simulink subsystem "GenCtrl"  (R2024b)
settings: Solver=VariableStepAuto  StartTime=0.0  StopTime=10.0  RelTol=1e-3
undefined symbols (not defined in the file or in its folder): SimIn, SimPar
libraries: simulink_extras x7, libAxisTransformations x3, ComponentsLib x3
settings Model: Creator=tbritton  LastModifiedBy=mjki1
settings SolverCC: AlgebraicLoopSolver=TrustRegion
settings OptimizationCC: ReuseModelBlockBuffer=off
settings DebuggingCC: UnconnectedInputMsg=warning  UnconnectedOutputMsg=warning  UnconnectedLineMsg=warning
settings ModelReferenceCC: EnableRefExpFcnMdlSchedulingChecks=on
settings RTWCC: GPUComputeCapability=3.5  DLArmComputeVersion=19.05

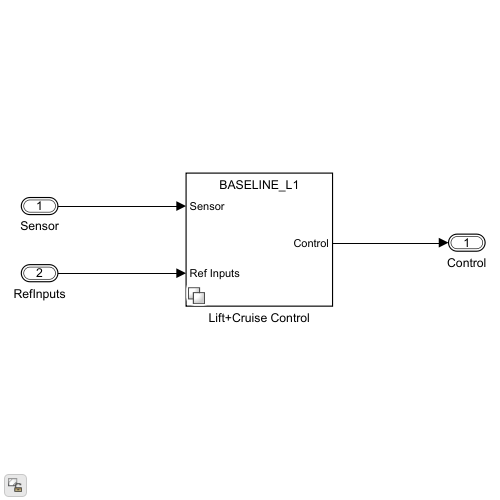
[thumbnail: Simulink's stored preview of the top-level diagram]
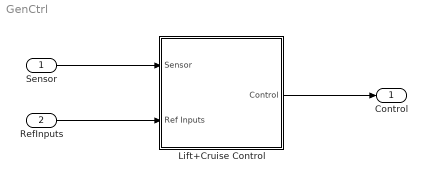
== system GenCtrl ==
  Sensor : Inport  OutDataTypeStr=Bus: SensorBus
  RefInputs : Inport  Port=2  OutDataTypeStr=Bus: BUS_REF_INPUT
  Lift+Cruise Control : Subsystem  Variant=on
  Control : Outport  OutDataTypeStr=Bus: BUS_CONTROL
  wires:
  Sensor/1 -> Lift+Cruise Control/1(Sensor)
  RefInputs/1 -> Lift+Cruise Control/2(Ref Inputs)
  Lift+Cruise Control/1(Control) -> Control/1

== system GenCtrl/Lift+Cruise Control ==
  Sensor : Inport  OutDataTypeStr=Bus: SensorBus
  Ref Inputs : Inport  Port=2  OutDataTypeStr=Bus: BUS_REF_INPUT
  BASELINE : Subsystem  VariantControl=GVS_CTRL_TYPE_BASELINE  ReferencedSubsystem=Baseline
  BASELINE_AGI : Subsystem  VariantControl=GVS_CTRL_TYPE_BASELINE_AGI  ReferencedSubsystem=BASELINE_AGI
  BASELINE_L1 : Subsystem  VariantControl=GVS_CTRL_TYPE_BASELINE_L1
  TRIM : Subsystem  VariantControl=GVS_CTRL_TYPE_TRIM  ReferencedSubsystem=TRIM
  Control : Outport  OutDataTypeStr=Bus: BUS_CONTROL  VectorParamsAs1DForOutWhenUnconnected=off

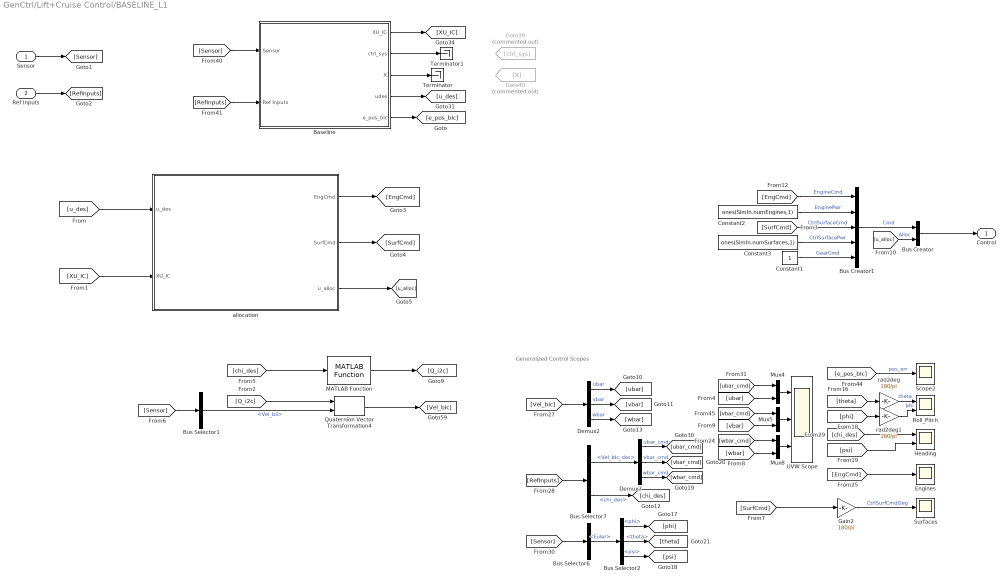
== system GenCtrl/Lift+Cruise Control/BASELINE_L1 ==
  note: Generalized Control Scopes
  Sensor : Inport  OutDataTypeStr=Bus: SensorBus
  Ref Inputs : Inport  Port=2  OutDataTypeStr=Bus: BUS_REF_INPUT
  Baseline : Subsystem
      settings: LibrarySourceBlock=ControllersLib/Baseline
  Bus Creator : BusCreator  Inputs=2
  Bus Creator1 : BusCreator  Inputs=5  OutDataTypeStr=Bus: BUS_CMD
  Bus Selector1 : BusSelector  OutputSignals=Vel_bIi
  Bus Selector2 : BusSelector  OutputSignals=phi,theta,psi
  Bus Selector6 : BusSelector  OutputSignals=Euler
  Bus Selector7 : BusSelector  OutputSignals=Vel_bIc_des,chi_des
  Constant1 : Constant
  Constant2 : Constant  Value=ones(SimIn.numEngines,1)
  Constant3 : Constant  Value=ones(SimIn.numSurfaces,1)
  Demux2 : Demux  Outputs=3
  Demux3 : Demux  Outputs=3
  Engines : Scope
  Gain2 : Gain  Gain=180/pi
  Goto39 : Goto  Commented=on  GotoTag=ctrl_sys
  Goto40 : Goto  Commented=on  GotoTag=X
  Heading : Scope  NumInputPorts=2
  MATLAB Function : ComponentsLib/ConvertToControlFrame/MATLAB Function  SystemSampleTime=-1  VariantActivationTime=update diagram  AllowFlexibleInterface=on  Latency=0  AutoFrameSizeCalculation=off
      settings: SourceProductName=Components
  Mux4 : Mux  Inputs=2
  Mux5 : Mux  Inputs=2
  Mux8 : Mux  Inputs=2
  Quaternion Vector Transformation4 : libAxisTransformations/Quaternion Vector Transformation  n=0
  Roll_Pitch : Scope  NumInputPorts=2
  Scope2 : Scope
  Surfaces : Scope
  Terminator : Terminator
  Terminator1 : Terminator
  UVW Scope : Scope  NumInputPorts=3
  allocation : Subsystem
  rad2deg : Gain  Gain=180/pi
  rad2deg1 : Gain  Gain=180/pi
  Control : Outport  OutDataTypeStr=Bus: BUS_CONTROL  VectorParamsAs1DForOutWhenUnconnected=off
  wires:
  Bus Creator/1 -> Control/1
  [u_alloc] -> Bus Creator/2  "Alloc"
  allocation/3(u_alloc) -> [u_alloc]
  allocation/2(SurfCmd) -> [SurfCmd]
  allocation/1(EngCmd) -> [EngCmd]
  [u_des] -> allocation/1(u_des)
  [XU_IC] -> allocation/2(XU_IC)
  [SurfCmd] -> Bus Creator1/3  "CtrlSurfaceCmd"
  Bus Creator1/1 -> Bus Creator/1  "Cmd"
  Constant3/1 -> Bus Creator1/4  "CtrlSurfacePwr"
  Constant1/1 -> Bus Creator1/5  "GearCmd"
  Constant2/1 -> Bus Creator1/2  "EnginePwr"
  [EngCmd] -> Bus Creator1/1  "EngineCmd"
  Baseline/1(XU_IC) -> [XU_IC]
  Baseline/5(e_pos_blc) -> [e_pos_bIc]
  Baseline/3(X) -> Terminator/1
  [Sensor] -> Baseline/1(Sensor)
  [RefInputs] -> Baseline/2(Ref Inputs)
  Baseline/4(udes) -> [u_des]
  Baseline/2(ctrl_sys) -> Terminator1/1
  Sensor/1 -> [Sensor]
  Ref Inputs/1 -> [RefInputs]
  MATLAB Function/1 -> [Q_i2c]
  Quaternion Vector Transformation4/1 -> [Vel_bIc]
  [Sensor] -> Bus Selector1/1
  Bus Selector1/1 -> Quaternion Vector Transformation4/2  "<Vel_bIi>"
  [Q_i2c] -> Quaternion Vector Transformation4/1
  [chi_des] -> MATLAB Function/1
  Demux3/2 -> [vbar_cmd]  "vbar_cmd"
  [Sensor] -> Bus Selector6/1
  Bus Selector7/1 -> Demux3/1  "<Vel_bIc_des>"
  Bus Selector2/2 -> [theta]  "<theta>"
  rad2deg/1 -> Roll_Pitch/1  "theta"
  [ubar_cmd] -> Mux4/1
  Mux4/1 -> UVW Scope/1
  Bus Selector6/1 -> Bus Selector2/1  "<Euler>"
  [e_pos_bIc] -> Scope2/1  "pos_err"
  Demux2/2 -> [vbar]  "vbar"
  [vbar] -> Mux5/2
  [wbar_cmd] -> Mux8/1
  [psi] -> Heading/2
  [phi] -> rad2deg1/1
  Bus Selector2/3 -> [psi]  "<psi>"
  Bus Selector7/2 -> [chi_des]  "<chi_des>"
  Mux5/1 -> UVW Scope/2
  Demux2/1 -> [ubar]  "ubar"
  Gain2/1 -> Surfaces/1  "CtrlSurfCmdDeg"
  [Vel_bIc] -> Demux2/1
  [wbar] -> Mux8/2
  [chi_des] -> Heading/1
  Demux2/3 -> [wbar]  "wbar"
  Mux8/1 -> UVW Scope/3
  [EngCmd] -> Engines/1
  [vbar_cmd] -> Mux5/1
  Demux3/3 -> [wbar_cmd]  "wbar_cmd"
  [SurfCmd] -> Gain2/1
  [ubar] -> Mux4/2
  Demux3/1 -> [ubar_cmd]  "ubar_cmd"
  rad2deg1/1 -> Roll_Pitch/2  "phi"
  [RefInputs] -> Bus Selector7/1
  Bus Selector2/1 -> [phi]  "<phi>"
  [theta] -> rad2deg/1

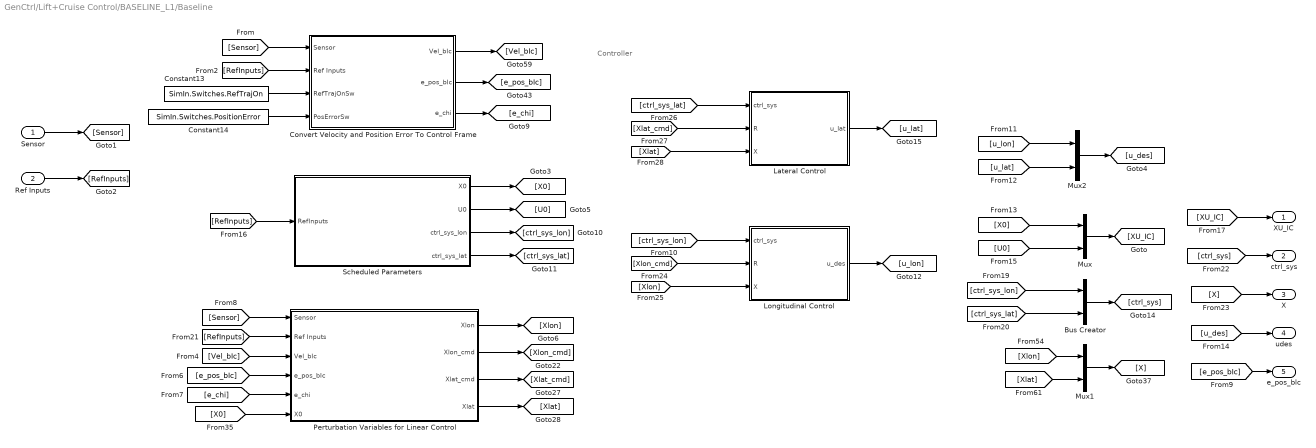
== system GenCtrl/Lift+Cruise Control/BASELINE_L1/Baseline ==
  note: Controller
  Sensor : Inport  OutDataTypeStr=Bus: SensorBus
  Ref Inputs : Inport  Port=2  OutDataTypeStr=Bus: BUS_REF_INPUT
  Bus Creator : BusCreator  Inputs=2
  Constant13 : Constant  Value=SimIn.Switches.RefTrajOn
  Constant14 : Constant  Value=SimIn.Switches.PositionError
  Convert Velocity and Position Error To Control Frame : Subsystem  AncestorBlock=ComponentsLib/ConvertToControlFrame
  Lateral Control : Subsystem
  Longitudinal Control : Subsystem
  Mux : Mux  Inputs=2
  Mux1 : Mux  Inputs=2
  Mux2 : Mux  Inputs=2
  Perturbation Variables for Linear Control : Subsystem  AncestorBlock=ComponentsLib/ComputePerturbationVariables
  Scheduled Parameters : Subsystem  AncestorBlock=ComponentsLib/FeedbackScheduling
      settings: LibrarySourceBlock=ComponentsLib/FeedbackScheduling
  XU_IC : Outport
  ctrl_sys : Outport  Port=2
  X : Outport  Port=3
  udes : Outport  Port=4
  e_pos_blc : Outport  Port=5
  wires:
  Mux2/1 -> [u_des]
  [u_lat] -> Mux2/2
  [u_lon] -> Mux2/1
  [e_pos_bIc] -> e_pos_blc/1
  [X0] -> Perturbation Variables for Linear Control/6(X0)
  Perturbation Variables for Linear Control/1(Xlon) -> [Xlon]
  [Sensor] -> Perturbation Variables for Linear Control/1(Sensor)
  Perturbation Variables for Linear Control/3(Xlat_cmd) -> [Xlat_cmd]
  Sensor/1 -> [Sensor]
  Scheduled Parameters/1(X0) -> [X0]
  Ref Inputs/1 -> [RefInputs]
  [RefInputs] -> Convert Velocity and Position Error To Control Frame/2(Ref Inputs)
  Convert Velocity and Position Error To Control Frame/1(Vel_bIc) -> [Vel_bIc]
  Convert Velocity and Position Error To Control Frame/2(e_pos_bIc) -> [e_pos_bIc]
  Scheduled Parameters/3(ctrl_sys_lon) -> [ctrl_sys_lon]
  [e_pos_bIc] -> Perturbation Variables for Linear Control/4(e_pos_bIc)
  Perturbation Variables for Linear Control/4(Xlat) -> [Xlat]
  [RefInputs] -> Scheduled Parameters/1(RefInputs)
  Perturbation Variables for Linear Control/2(Xlon_cmd) -> [Xlon_cmd]
  Convert Velocity and Position Error To Control Frame/3(e_chi) -> [e_chi]
  [Sensor] -> Convert Velocity and Position Error To Control Frame/1(Sensor)
  [Vel_bIc] -> Perturbation Variables for Linear Control/3(Vel_bIc)
  Constant13/1 -> Convert Velocity and Position Error To Control Frame/3(RefTrajOnSw)
  [RefInputs] -> Perturbation Variables for Linear Control/2(Ref Inputs)
  Constant14/1 -> Convert Velocity and Position Error To Control Frame/4(PosErrorSw)
  [e_chi] -> Perturbation Variables for Linear Control/5(e_chi)
  Scheduled Parameters/2(U0) -> [U0]
  Scheduled Parameters/4(ctrl_sys_lat) -> [ctrl_sys_lat]
  [u_des] -> udes/1
  [X0] -> Mux/1
  [U0] -> Mux/2
  Mux/1 -> [XU_IC]
  [XU_IC] -> XU_IC/1
  [ctrl_sys_lon] -> Bus Creator/1
  [ctrl_sys_lat] -> Bus Creator/2
  Bus Creator/1 -> [ctrl_sys]
  [ctrl_sys] -> ctrl_sys/1
  Mux1/1 -> [X]
  [Xlon] -> Mux1/1
  [Xlat] -> Mux1/2
  [X] -> X/1
  [ctrl_sys_lon] -> Longitudinal Control/1(ctrl_sys)
  [Xlon_cmd] -> Longitudinal Control/2(R)
  [Xlon] -> Longitudinal Control/3(X)
  Longitudinal Control/1(u_des) -> [u_lon]
  Lateral Control/1(u_lat) -> [u_lat]
  [Xlat_cmd] -> Lateral Control/2(R)
  [Xlat] -> Lateral Control/3(X)
  [ctrl_sys_lat] -> Lateral Control/1(ctrl_sys)

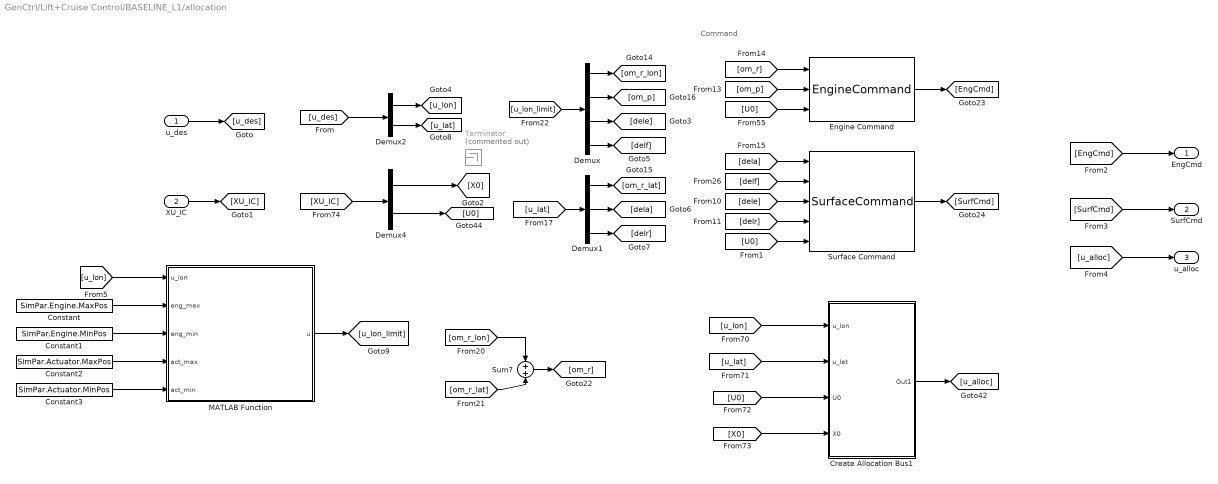
== system GenCtrl/Lift+Cruise Control/BASELINE_L1/allocation ==
  note: Command
  u_des : Inport
  XU_IC : Inport  Port=2
  Constant : Constant  Value=SimPar.Engine.MaxPos
  Constant1 : Constant  Value=SimPar.Engine.MinPos
  Constant2 : Constant  Value=SimPar.Actuator.MaxPos
  Constant3 : Constant  Value=SimPar.Actuator.MinPos
  Create Allocation Bus1 : Subsystem  AncestorBlock=ComponentsLib/CreateAllocationBus
  Demux : Demux  Outputs=[8 1 1 1]
  Demux1 : Demux  Outputs=[8 1 1]
  Demux2 : Demux  Outputs=[11 10]
  Demux4 : Demux  Outputs=[12 13]
  Engine Command : ComponentsLib/EngineCommand  SystemSampleTime=-1  VariantActivationTime=update diagram  AllowFlexibleInterface=on  Latency=0  AutoFrameSizeCalculation=off
      settings: SourceProductName=Components
  MATLAB Function : MATLAB Function  TreatAsAtomicUnit=on
  Sum7 : Sum
  Surface Command : ComponentsLib/SurfaceCommand  SystemSampleTime=-1  VariantActivationTime=update diagram  AllowFlexibleInterface=on  Latency=0  AutoFrameSizeCalculation=off
      settings: SourceProductName=Components
  Terminator : Terminator  Commented=on
  EngCmd : Outport
  SurfCmd : Outport  Port=2
  u_alloc : Outport  Port=3
  wires:
  Constant3/1 -> MATLAB Function/5(act_min)
  Constant2/1 -> MATLAB Function/4(act_max)
  Constant1/1 -> MATLAB Function/3(eng_min)
  Constant/1 -> MATLAB Function/2(eng_max)
  [u_lon] -> MATLAB Function/1(u_lon)
  MATLAB Function/1(u) -> [u_lon_limit]
  [u_alloc] -> u_alloc/1
  [EngCmd] -> EngCmd/1
  [SurfCmd] -> SurfCmd/1
  u_des/1 -> [u_des]
  XU_IC/1 -> [XU_IC]
  [u_lon] -> Create Allocation Bus1/1(u_lon)
  [U0] -> Create Allocation Bus1/3(U0)
  [X0] -> Create Allocation Bus1/4(X0)
  [u_lat] -> Create Allocation Bus1/2(u_lat)
  Create Allocation Bus1/1(Out1) -> [u_alloc]
  Surface Command/1 -> [SurfCmd]
  Demux1/1 -> [om_r_lat]
  [om_r] -> Engine Command/1
  [om_p] -> Engine Command/2
  [XU_IC] -> Demux4/1
  [U0] -> Engine Command/3
  Demux1/2 -> [dela]
  [U0] -> Surface Command/5
  [dele] -> Surface Command/3
  [delr] -> Surface Command/4
  Demux/3 -> [dele]
  Demux/1 -> [om_r_lon]
  Demux/2 -> [om_p]
  Demux1/3 -> [delr]
  [u_des] -> Demux2/1
  [delf] -> Surface Command/2
  Demux4/1 -> [X0]
  Demux4/2 -> [U0]
  [u_lat] -> Demux1/1
  Demux2/1 -> [u_lon]
  Demux2/2 -> [u_lat]
  [u_lon_limit] -> Demux/1
  [dela] -> Surface Command/1
  Engine Command/1 -> [EngCmd]
  Demux/4 -> [delf]
  [om_r_lon] -> Sum7/1
  [om_r_lat] -> Sum7/2
  Sum7/1 -> [om_r]

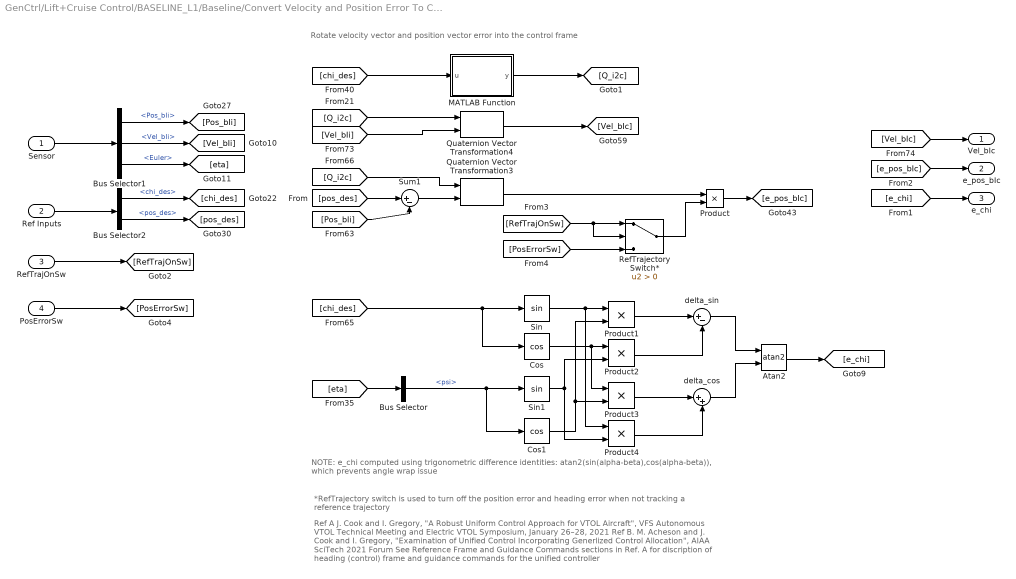
== system GenCtrl/Lift+Cruise Control/BASELINE_L1/Baseline/Convert Velocity and Position Error To Control Frame ==
  note: NOTE: e_chi computed using trigonometric difference identities: atan2(sin(alpha-beta),cos(alpha-beta)), which prevents angle wrap issue
  note: *RefTrajectory switch is used to turn off the position error and heading error when not tracking a reference trajectory
  note: Ref A
      | J. Cook and I. Gregory, "A Robust Uniform Control Approach for VTOL Aircraft", VFS Autonomous VTOL Technical Meeting and Electric VTOL Symposium, January 26–28, 2021
      |
      | Ref B.
      | M. Acheson and J. Cook and I. Gregory, "Examination of Unified Control Incorporating Generlized Control Allocation", AIAA SciTech 2021 Forum
      |
      | See Reference Frame and Guidance Commands sections in Ref. A for discription of heading (control) frame and guidance commands for the unified controller
  note: Rotate velocity vector and position vector error into the control frame
  Sensor : Inport  OutDataTypeStr=Bus: SensorBus
  Ref Inputs : Inport  Port=2  OutDataTypeStr=Bus: BUS_REF_INPUT
  RefTrajOnSw : Inport  Port=3
  PosErrorSw : Inport  Port=4
  Atan2 : Trigonometry  Operator=atan2
  Bus Selector : BusSelector  OutputSignals=psi
  Bus Selector1 : BusSelector  OutputSignals=Pos_bIi,Vel_bIi,Euler
  Bus Selector2 : BusSelector  OutputSignals=chi_des,pos_des
  Cos : Trigonometry  Operator=cos
  Cos1 : Trigonometry  Operator=cos
  MATLAB Function : MATLAB Function  TreatAsAtomicUnit=on
  Product{,1..4} (5 alike) : Product
  Quaternion Vector Transformation3 : libAxisTransformations/Quaternion Vector Transformation  n=0
  Quaternion Vector Transformation4 : libAxisTransformations/Quaternion Vector Transformation  n=0
  RefTrajectory Switch* : Switch  Criteria=u2 > Threshold  SaturateOnIntegerOverflow=off  InputSameDT=off
  Sin : Trigonometry
  Sin1 : Trigonometry
  Sum1 : Sum  Inputs=|+-
  delta_cos : Sum  Inputs=|++
  delta_sin : Sum  Inputs=|+-
  Vel_bIc : Outport
  e_pos_bIc : Outport  Port=2
  e_chi : Outport  Port=3
  wires:
  Sensor/1 -> Bus Selector1/1
  Quaternion Vector Transformation4/1 -> [Vel_bIc]
  [chi_des] -> Cos/1, Sin/1
  Sum1/1 -> Quaternion Vector Transformation3/2
  [e_pos_bIc] -> e_pos_bIc/1
  RefTrajOnSw/1 -> [RefTrajOnSw]
  Bus Selector2/1 -> [chi_des]  "<chi_des>"
  Bus Selector1/2 -> [Vel_bIi]  "<Vel_bIi>"
  PosErrorSw/1 -> [PosErrorSw]
  [Vel_bIi] -> Quaternion Vector Transformation4/2
  Atan2/1 -> [e_chi]
  Bus Selector1/1 -> [Pos_bIi]  "<Pos_bIi>"
  Bus Selector2/2 -> [pos_des]  "<pos_des>"
  [RefTrajOnSw] -> RefTrajectory Switch*/1, RefTrajectory Switch*/2
  [Vel_bIc] -> Vel_bIc/1
  [Pos_bIi] -> Sum1/2
  RefTrajectory Switch*/1 -> Product/2
  [chi_des] -> MATLAB Function/1(u)
  [e_chi] -> e_chi/1
  [pos_des] -> Sum1/1
  Quaternion Vector Transformation3/1 -> Product/1
  [Q_i2c] -> Quaternion Vector Transformation3/1
  Product/1 -> [e_pos_bIc]
  Ref Inputs/1 -> Bus Selector2/1
  MATLAB Function/1(y) -> [Q_i2c]
  Bus Selector1/3 -> [eta]  "<Euler>"
  [PosErrorSw] -> RefTrajectory Switch*/3
  [eta] -> Bus Selector/1
  [Q_i2c] -> Quaternion Vector Transformation4/1
  Bus Selector/1 -> Cos1/1, Sin1/1  "<psi>"
  Sin/1 -> Product1/1, Product4/1
  Cos/1 -> Product3/1, Product2/1
  Sin1/1 -> Product4/2, Product2/2
  Cos1/1 -> Product3/2, Product1/2
  Product1/1 -> delta_sin/1
  Product2/1 -> delta_sin/2
  Product3/1 -> delta_cos/1
  Product4/1 -> delta_cos/2
  delta_sin/1 -> Atan2/1
  delta_cos/1 -> Atan2/2

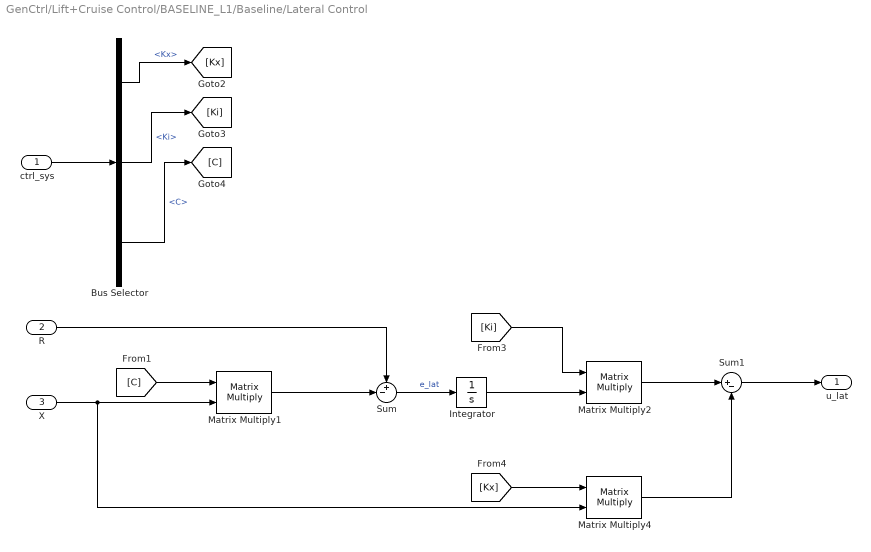
== system GenCtrl/Lift+Cruise Control/BASELINE_L1/Baseline/Lateral Control ==
  ctrl_sys : Inport
  R : Inport  Port=2
  X : Inport  Port=3
  Bus Selector : BusSelector  OutputSignals=Kx,Ki,C
  Integrator : Integrator
  Matrix Multiply1 : Product  Multiplication=Matrix(*)
  Matrix Multiply2 : Product  Multiplication=Matrix(*)
  Matrix Multiply4 : Product  Multiplication=Matrix(*)
  Sum : Sum  Inputs=+-|
  Sum1 : Sum  Inputs=|+-
  u_lat : Outport
  wires:
  Matrix Multiply4/1 -> Sum1/2
  Matrix Multiply2/1 -> Sum1/1
  ctrl_sys/1 -> Bus Selector/1
  Bus Selector/1 -> [Kx]  "<Kx>"
  Bus Selector/2 -> [Ki]  "<Ki>"
  Bus Selector/3 -> [C]  "<C>"
  R/1 -> Sum/1
  [C] -> Matrix Multiply1/1
  X/1 -> Matrix Multiply1/2, Matrix Multiply4/2
  Matrix Multiply1/1 -> Sum/2
  [Ki] -> Matrix Multiply2/1
  Sum/1 -> Integrator/1  "e_lat"
  Integrator/1 -> Matrix Multiply2/2
  [Kx] -> Matrix Multiply4/1
  Sum1/1 -> u_lat/1

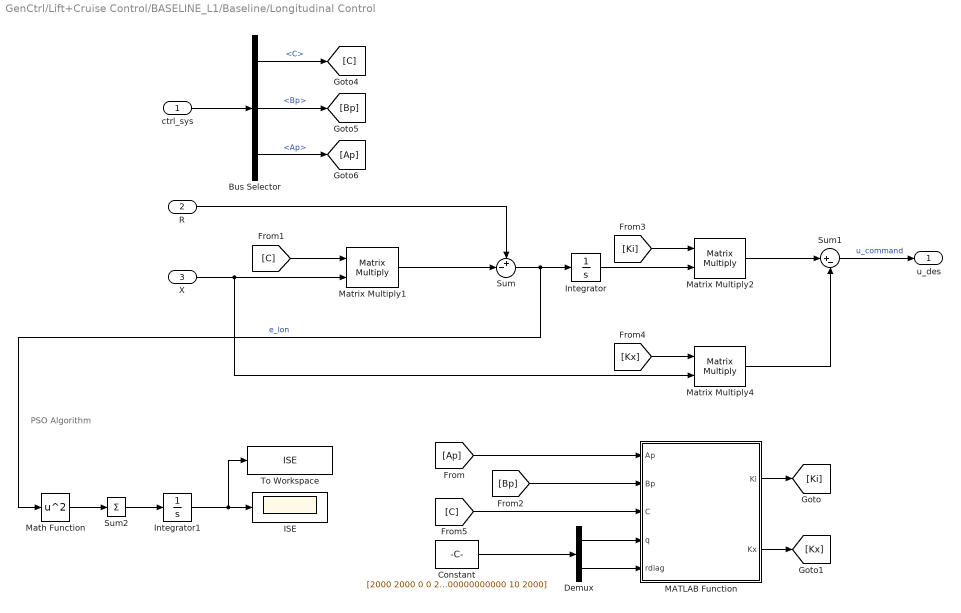
== system GenCtrl/Lift+Cruise Control/BASELINE_L1/Baseline/Longitudinal Control ==
  note: PSO Algorithm
  ctrl_sys : Inport
  R : Inport  Port=2
  X : Inport  Port=3
  Bus Selector : BusSelector  OutputSignals=C,Bp,Ap
  Constant : Constant  Value="[2000\t2000\t0\t0\t2000\t0 2000\t0.00100000000000000\t0.00100000000000000\t1193.13747312064\t2000\t646.275872645163\t0.00100000000000000\t2000\t0.00100000000000000\t10\t2000]"
  Demux : Demux  Outputs=[6 11]
  ISE : Scope
  Integrator : Integrator
  Integrator1 : Integrator
  MATLAB Function : MATLAB Function  TreatAsAtomicUnit=on
  Math Function : Math  Operator=square
  Matrix Multiply1 : Product  Multiplication=Matrix(*)
  Matrix Multiply2 : Product  Multiplication=Matrix(*)
  Matrix Multiply4 : Product  Multiplication=Matrix(*)
  Sum : Sum  Inputs=+-|
  Sum1 : Sum  Inputs=|+-
  Sum2 : Sum  Inputs=+
  To Workspace : ToWorkspace  VariableName=ISE  SampleTime=-1
      settings: Save2DSignal=2-D array (concatenate along first dimension)
  u_des : Outport
  wires:
  Demux/2 -> MATLAB Function/5(rdiag)
  Demux/1 -> MATLAB Function/4(q)
  Constant/1 -> Demux/1
  Bus Selector/3 -> [Ap]  "<Ap>"
  Bus Selector/2 -> [Bp]  "<Bp>"
  MATLAB Function/2(Kx) -> [Kx]
  [Ap] -> MATLAB Function/1(Ap)
  [C] -> MATLAB Function/3(C)
  [Bp] -> MATLAB Function/2(Bp)
  MATLAB Function/1(Ki) -> [Ki]
  Sum/1 -> Integrator/1, Math Function/1  "e_lon"
  Sum2/1 -> Integrator1/1
  Math Function/1 -> Sum2/1
  Integrator1/1 -> ISE/1, To Workspace/1
  Matrix Multiply4/1 -> Sum1/2
  Matrix Multiply2/1 -> Sum1/1
  ctrl_sys/1 -> Bus Selector/1
  Bus Selector/1 -> [C]  "<C>"
  R/1 -> Sum/1
  [C] -> Matrix Multiply1/1
  X/1 -> Matrix Multiply1/2, Matrix Multiply4/2
  Matrix Multiply1/1 -> Sum/2
  [Ki] -> Matrix Multiply2/1
  Integrator/1 -> Matrix Multiply2/2
  [Kx] -> Matrix Multiply4/1
  Sum1/1 -> u_des/1  "u_command"

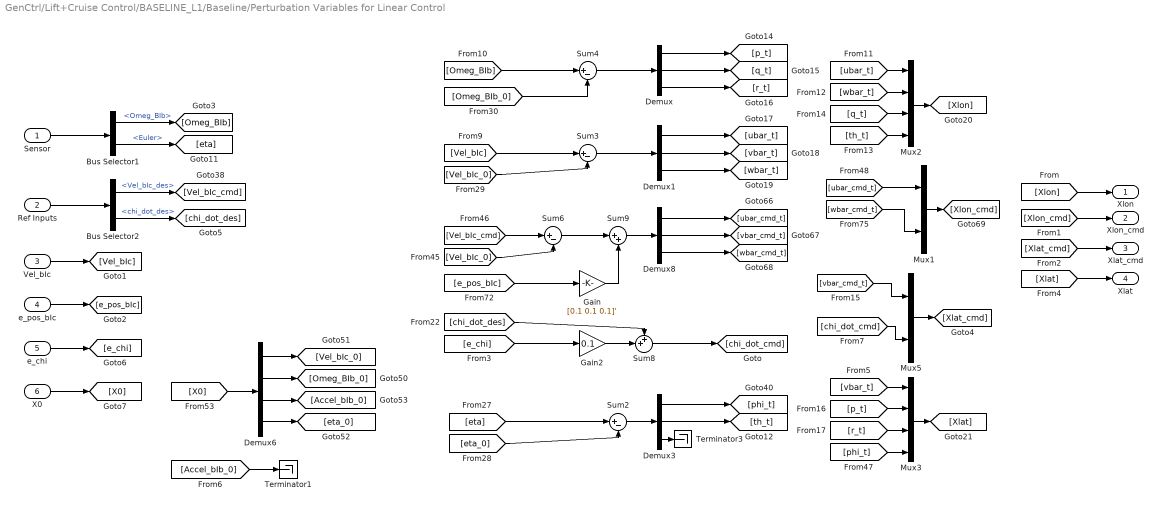
== system GenCtrl/Lift+Cruise Control/BASELINE_L1/Baseline/Perturbation Variables for Linear Control ==
  Sensor : Inport  OutDataTypeStr=Bus: SensorBus
  Ref Inputs : Inport  Port=2  OutDataTypeStr=Bus: BUS_REF_INPUT
  Vel_bIc : Inport  Port=3
  e_pos_bIc : Inport  Port=4
  e_chi : Inport  Port=5
  X0 : Inport  Port=6
  Bus Selector1 : BusSelector  OutputSignals=Omeg_BIb,Euler
  Bus Selector2 : BusSelector  OutputSignals=Vel_bIc_des,chi_dot_des
  Demux{,1,3,8} (4 alike) : Demux  Outputs=3
  Demux6 : Demux  Outputs=[3 3 3 3]
  Gain : Gain  Gain=[0.1 0.1 0.1]'
  Gain2 : Gain  Gain=0.1
  Mux1 : Mux  Inputs=2
  Mux2 : Mux
  Mux3 : Mux
  Mux5 : Mux  Inputs=2
  Sum{2..4,6} (4 alike) : Sum  Inputs=|+-
  Sum8 : Sum  Inputs=++|
  Sum9 : Sum  Inputs=|++
  Terminator1 : Terminator
  Terminator3 : Terminator
  Xlon : Outport
  Xlon_cmd : Outport  Port=2
  Xlat_cmd : Outport  Port=3
  Xlat : Outport  Port=4
  wires:
  [Omeg_BIb_0] -> Sum4/2
  Sum9/1 -> Demux8/1
  [Vel_bIc] -> Sum3/1
  [Vel_bIc_0] -> Sum3/2
  [chi_dot_cmd] -> Mux5/2
  Demux1/1 -> [ubar_t]
  [eta] -> Sum2/1
  Demux3/2 -> [th_t]
  Demux3/3 -> Terminator3/1
  Demux3/1 -> [phi_t]
  Demux1/3 -> [wbar_t]
  Demux/1 -> [p_t]
  Gain2/1 -> Sum8/2
  Mux2/1 -> [Xlon]
  Sum8/1 -> [chi_dot_cmd]
  [e_chi] -> Gain2/1
  [Vel_bIc_0] -> Sum6/2
  [r_t] -> Mux3/3
  [vbar_cmd_t] -> Mux5/1
  Gain/1 -> Sum9/2
  [ubar_t] -> Mux2/1
  Mux5/1 -> [Xlat_cmd]
  [q_t] -> Mux2/3
  Demux1/2 -> [vbar_t]
  [chi_dot_des] -> Sum8/1
  Mux1/1 -> [Xlon_cmd]
  [vbar_t] -> Mux3/1
  [wbar_cmd_t] -> Mux1/2
  [e_pos_bIc] -> Gain/1
  Demux8/3 -> [wbar_cmd_t]
  [phi_t] -> Mux3/4
  Demux8/1 -> [ubar_cmd_t]
  Sum6/1 -> Sum9/1
  [Vel_bIc_cmd] -> Sum6/1
  Demux8/2 -> [vbar_cmd_t]
  Sum2/1 -> Demux3/1
  Demux/3 -> [r_t]
  Sum3/1 -> Demux1/1
  Sum4/1 -> Demux/1
  Mux3/1 -> [Xlat]
  [p_t] -> Mux3/2
  [th_t] -> Mux2/4
  Demux/2 -> [q_t]
  [ubar_cmd_t] -> Mux1/1
  [wbar_t] -> Mux2/2
  [eta_0] -> Sum2/2
  [Omeg_BIb] -> Sum4/1
  [Xlon] -> Xlon/1
  [Xlon_cmd] -> Xlon_cmd/1
  [Xlat_cmd] -> Xlat_cmd/1
  [Xlat] -> Xlat/1
  Bus Selector1/2 -> [eta]  "<Euler>"
  Sensor/1 -> Bus Selector1/1
  Bus Selector1/1 -> [Omeg_BIb]  "<Omeg_BIb>"
  Vel_bIc/1 -> [Vel_bIc]
  Ref Inputs/1 -> Bus Selector2/1
  Bus Selector2/1 -> [Vel_bIc_cmd]  "<Vel_bIc_des>"
  Bus Selector2/2 -> [chi_dot_des]  "<chi_dot_des>"
  e_pos_bIc/1 -> [e_pos_bIc]
  e_chi/1 -> [e_chi]
  Demux6/1 -> [Vel_bIc_0]
  Demux6/3 -> [Accel_bIb_0]
  [X0] -> Demux6/1
  Demux6/4 -> [eta_0]
  Demux6/2 -> [Omeg_BIb_0]
  X0/1 -> [X0]
  [Accel_bIb_0] -> Terminator1/1

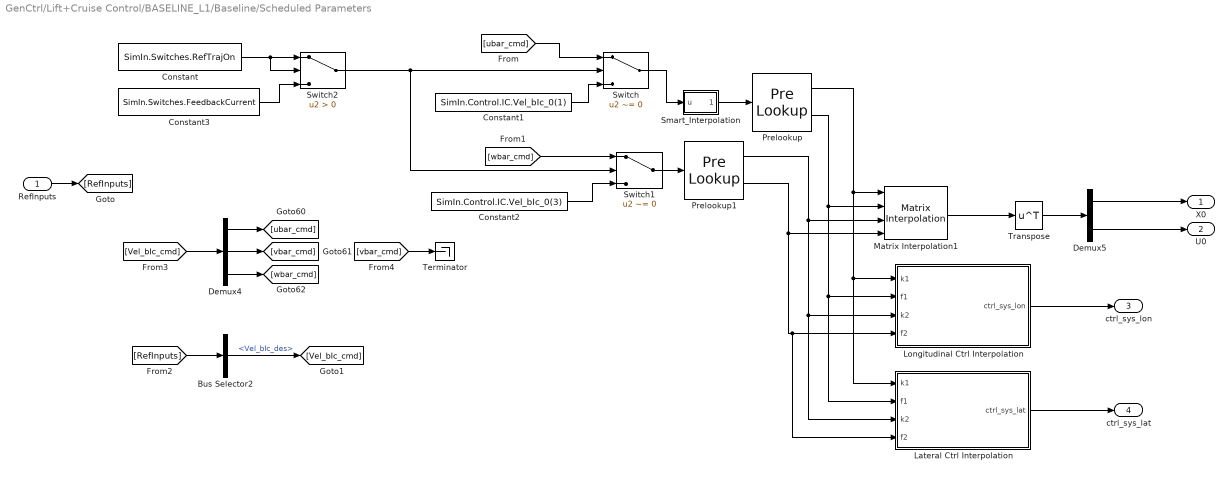
== system GenCtrl/Lift+Cruise Control/BASELINE_L1/Baseline/Scheduled Parameters ==
  RefInputs : Inport  OutDataTypeStr=Bus: BUS_REF_INPUT
  Bus Selector2 : BusSelector  OutputSignals=Vel_bIc_des
  Constant : Constant  Value=SimIn.Switches.RefTrajOn
  Constant1 : Constant  Value=SimIn.Control.IC.Vel_bIc_0(1)
  Constant2 : Constant  Value=SimIn.Control.IC.Vel_bIc_0(3)
  Constant3 : Constant  Value=SimIn.Switches.FeedbackCurrent
  Demux4 : Demux  Outputs=3
  Demux5 : Demux  Outputs=[12 13]
  Lateral Ctrl Interpolation : Subsystem
  Longitudinal Ctrl Interpolation : Subsystem
  Matrix Interpolation1 : simulink_extras/Additional Lookup Tables/Matrix Interpolation  InterpMethod=Linear  ExtrapMethod=Clip  InterpolateDimension=2  TableData=SimIn.Control.trim.XU0_interp  SimulateUsing=Code generation
  Prelookup : PreLookup  BreakpointsData=SimIn.Control.trim.UH
  Prelookup1 : PreLookup  BreakpointsData=SimIn.Control.trim.WH
  Smart_Interpolation : MATLAB Function  TreatAsAtomicUnit=on
  Switch : Switch  Criteria=u2 ~= 0  SaturateOnIntegerOverflow=off  InputSameDT=off
  Switch1 : Switch  Criteria=u2 ~= 0  SaturateOnIntegerOverflow=off  InputSameDT=off
  Switch2 : Switch  Criteria=u2 > Threshold  SaturateOnIntegerOverflow=off  InputSameDT=off
  Terminator : Terminator
  Transpose : Math  Operator=transpose
  X0 : Outport
  U0 : Outport  Port=2
  ctrl_sys_lon : Outport  Port=3
  ctrl_sys_lat : Outport  Port=4
  wires:
  Prelookup/1 -> Lateral Ctrl Interpolation/1(k1), Longitudinal Ctrl Interpolation/1(k1), Matrix Interpolation1/1
  Prelookup/2 -> Matrix Interpolation1/2, Lateral Ctrl Interpolation/2(f1), Longitudinal Ctrl Interpolation/2(f1)
  Smart_Interpolation/1(u_out) -> Prelookup/1
  Switch/1 -> Smart_Interpolation/1(u)
  Constant3/1 -> Switch2/3
  Constant/1 -> Switch2/2, Switch2/1
  Switch2/1 -> Switch/2, Switch1/2
  Constant2/1 -> Switch1/3
  Switch1/1 -> Prelookup1/1
  Constant1/1 -> Switch/3
  Longitudinal Ctrl Interpolation/1(ctrl_sys_lon) -> ctrl_sys_lon/1
  Lateral Ctrl Interpolation/1(ctrl_sys_lat) -> ctrl_sys_lat/1
  Prelookup1/2 -> Matrix Interpolation1/4, Lateral Ctrl Interpolation/4(f2), Longitudinal Ctrl Interpolation/4(f2)
  Prelookup1/1 -> Matrix Interpolation1/3, Lateral Ctrl Interpolation/3(k2), Longitudinal Ctrl Interpolation/3(k2)
  Demux5/2 -> U0/1
  Demux5/1 -> X0/1
  Transpose/1 -> Demux5/1
  Matrix Interpolation1/1 -> Transpose/1
  Demux4/1 -> [ubar_cmd]
  Demux4/3 -> [wbar_cmd]
  Demux4/2 -> [vbar_cmd]
  [Vel_bIc_cmd] -> Demux4/1
  RefInputs/1 -> [RefInputs]
  [ubar_cmd] -> Switch/1
  [RefInputs] -> Bus Selector2/1
  Bus Selector2/1 -> [Vel_bIc_cmd]  "<Vel_bIc_des>"
  [vbar_cmd] -> Terminator/1
  [wbar_cmd] -> Switch1/1

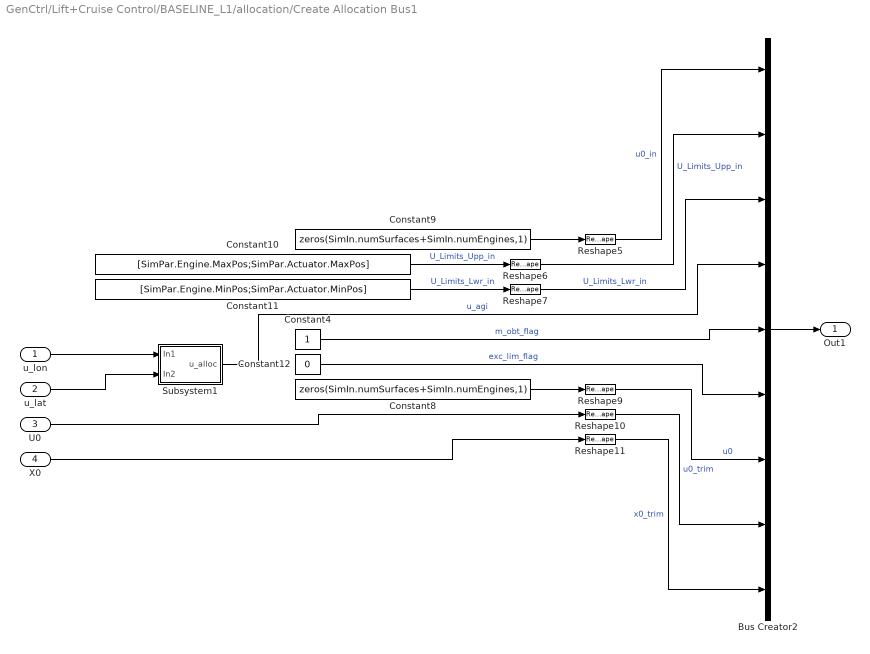
== system GenCtrl/Lift+Cruise Control/BASELINE_L1/allocation/Create Allocation Bus1 ==
  u_lon : Inport
  u_lat : Inport  Port=2
  U0 : Inport  Port=3
  X0 : Inport  Port=4
  Bus Creator2 : BusCreator  Inputs=9  OutDataTypeStr=Bus: BUS_ALLOC
  Constant10 : Constant  Value=[SimPar.Engine.MaxPos;SimPar.Actuator.MaxPos]
  Constant11 : Constant  Value=[SimPar.Engine.MinPos;SimPar.Actuator.MinPos]
  Constant12 : Constant  Value=0
  Constant4 : Constant
  Constant8 : Constant  Value=zeros(SimIn.numSurfaces+SimIn.numEngines,1)
  Constant9 : Constant  Value=zeros(SimIn.numSurfaces+SimIn.numEngines,1)
  Reshape{5..7,9..11} (6 alike) : Reshape
  Subsystem1 : Subsystem
  Out1 : Outport
  wires:
  Reshape7/1 -> Bus Creator2/3  "U_Limits_Lwr_in"
  Reshape5/1 -> Bus Creator2/1  "u0_in"
  Constant10/1 -> Reshape6/1  "U_Limits_Upp_in"
  u_lat/1 -> Subsystem1/2(In2)
  Constant12/1 -> Bus Creator2/6  "exc_lim_flag"
  Constant9/1 -> Reshape5/1
  Constant11/1 -> Reshape7/1  "U_Limits_Lwr_in"
  Reshape10/1 -> Bus Creator2/8  "u0_trim"
  Constant8/1 -> Reshape9/1
  U0/1 -> Reshape10/1
  Constant4/1 -> Bus Creator2/5  "m_obt_flag"
  Subsystem1/1(u_alloc) -> Bus Creator2/4  "u_agi"
  Reshape9/1 -> Bus Creator2/7  "u0"
  Reshape11/1 -> Bus Creator2/9  "x0_trim"
  Reshape6/1 -> Bus Creator2/2  "U_Limits_Upp_in"
  u_lon/1 -> Subsystem1/1(In1)
  X0/1 -> Reshape11/1
  Bus Creator2/1 -> Out1/1

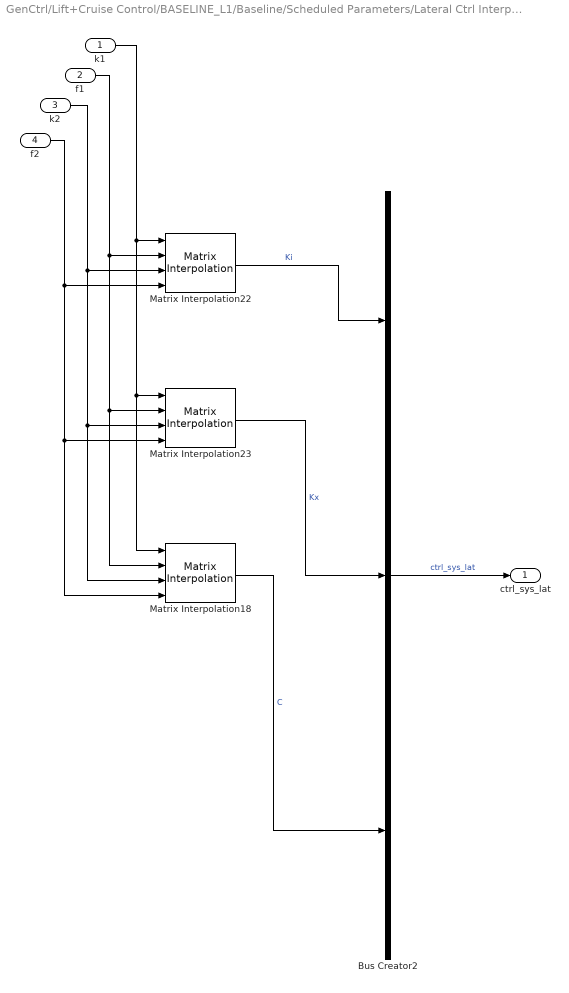
== system GenCtrl/Lift+Cruise Control/BASELINE_L1/Baseline/Scheduled Parameters/Lateral Ctrl Interpolation ==
  k1 : Inport
  f1 : Inport  Port=2
  k2 : Inport  Port=3
  f2 : Inport  Port=4
  Bus Creator2 : BusCreator  Inputs=3
  Matrix Interpolation18 : simulink_extras/Additional Lookup Tables/Matrix Interpolation  InterpMethod=Linear  ExtrapMethod=Clip  InterpolateDimension=2  TableData=SimIn.Control.trim.C_lat_interp  SimulateUsing=Code generation
  Matrix Interpolation22 : simulink_extras/Additional Lookup Tables/Matrix Interpolation  InterpMethod=Linear  ExtrapMethod=Clip  InterpolateDimension=2  TableData=SimIn.Control.trim.Ki_lat_interp  SimulateUsing=Code generation
  Matrix Interpolation23 : simulink_extras/Additional Lookup Tables/Matrix Interpolation  InterpMethod=Linear  ExtrapMethod=Clip  InterpolateDimension=2  TableData=SimIn.Control.trim.Kx_lat_interp  SimulateUsing=Code generation
  ctrl_sys_lat : Outport
  wires:
  Matrix Interpolation18/1 -> Bus Creator2/3  "C"
  Bus Creator2/1 -> ctrl_sys_lat/1  "ctrl_sys_lat"
  Matrix Interpolation23/1 -> Bus Creator2/2  "Kx"
  Matrix Interpolation22/1 -> Bus Creator2/1  "Ki"
  f1/1 -> Matrix Interpolation18/2, Matrix Interpolation23/2, Matrix Interpolation22/2
  f2/1 -> Matrix Interpolation18/4, Matrix Interpolation23/4, Matrix Interpolation22/4
  k2/1 -> Matrix Interpolation18/3, Matrix Interpolation23/3, Matrix Interpolation22/3
  k1/1 -> Matrix Interpolation18/1, Matrix Interpolation23/1, Matrix Interpolation22/1

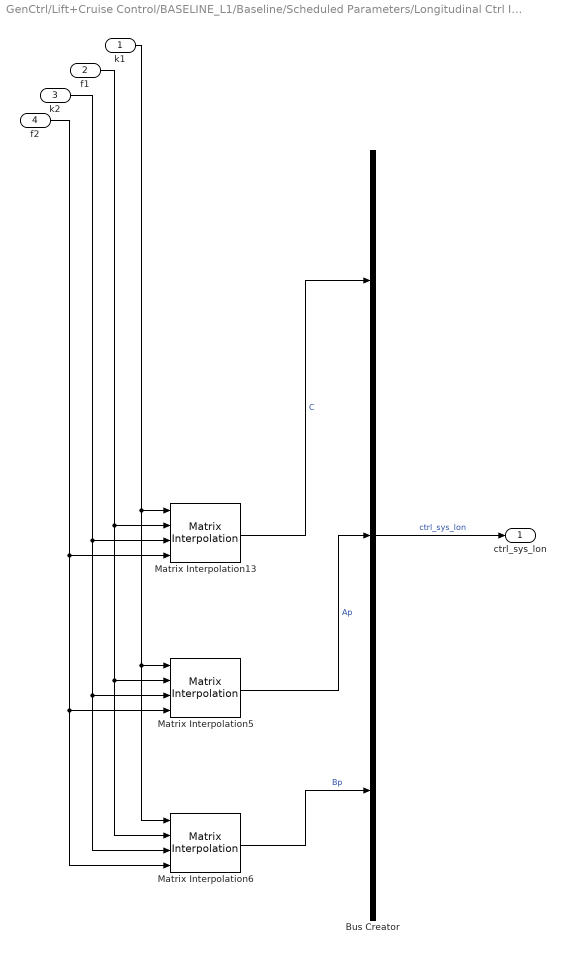
== system GenCtrl/Lift+Cruise Control/BASELINE_L1/Baseline/Scheduled Parameters/Longitudinal Ctrl Interpolation ==
  k1 : Inport
  f1 : Inport  Port=2
  k2 : Inport  Port=3
  f2 : Inport  Port=4
  Bus Creator : BusCreator  Inputs=3
  Matrix Interpolation13 : simulink_extras/Additional Lookup Tables/Matrix Interpolation  InterpMethod=Linear  ExtrapMethod=Clip  InterpolateDimension=2  TableData=SimIn.Control.trim.C_lon_interp  SimulateUsing=Code generation
  Matrix Interpolation5 : simulink_extras/Additional Lookup Tables/Matrix Interpolation  InterpMethod=Linear  ExtrapMethod=Clip  InterpolateDimension=2  TableData=SimIn.Control.trim.Ap_lon_interp  SimulateUsing=Code generation
  Matrix Interpolation6 : simulink_extras/Additional Lookup Tables/Matrix Interpolation  InterpMethod=Linear  ExtrapMethod=Clip  InterpolateDimension=2  TableData=SimIn.Control.trim.Bp_lon_interp  SimulateUsing=Code generation
  ctrl_sys_lon : Outport
  wires:
  Matrix Interpolation13/1 -> Bus Creator/1  "C"
  Bus Creator/1 -> ctrl_sys_lon/1  "ctrl_sys_lon"
  f2/1 -> Matrix Interpolation13/4, Matrix Interpolation5/4, Matrix Interpolation6/4
  Matrix Interpolation5/1 -> Bus Creator/2  "Ap"
  k1/1 -> Matrix Interpolation13/1, Matrix Interpolation5/1, Matrix Interpolation6/1
  k2/1 -> Matrix Interpolation13/3, Matrix Interpolation5/3, Matrix Interpolation6/3
  Matrix Interpolation6/1 -> Bus Creator/3  "Bp"
  f1/1 -> Matrix Interpolation13/2, Matrix Interpolation5/2, Matrix Interpolation6/2

== system GenCtrl/Lift+Cruise Control/BASELINE_L1/allocation/Create Allocation Bus1/Subsystem1 ==
  In1 : Inport
  In2 : Inport  Port=2
  Demux2 : Demux  Outputs=[8 1 1 1]
  Demux9 : Demux  Outputs=[8 1 1]
  Gain : Gain  Gain=-1
  Mux9 : Mux  Inputs=7
  Sum : Sum  Inputs=|++
  Terminator : Terminator
  u_alloc : Outport
  wires:
  Gain/1 -> Mux9/4  "dela"
  In1/1 -> Demux2/1
  Mux9/1 -> u_alloc/1  "u_alloc"
  Demux9/2 -> Mux9/3, Gain/1  "dela"
  Demux2/1 -> Sum/1  "om_r"
  Sum/1 -> Mux9/1  "om_r"
  Demux2/2 -> Mux9/2  "om_p"
  Demux2/3 -> Mux9/6, Mux9/5  "dele"
  Demux2/4 -> Terminator/1  "delf"
  In2/1 -> Demux9/1
  Demux9/3 -> Mux9/7  "delr"
  Demux9/1 -> Sum/2  "om_r"

== matlab function GenCtrl/Lift+Cruise Control/BASELINE_L1/Baseline/Convert Velocity and Position Error To Control Frame/MATLAB Function ==
  data: u input; y output double size=[4,1]
function y = fcn(u)

s = cos(u/2);
v = sin(u/2);
y = [s, 0*v, 0*v, v]';

== matlab function GenCtrl/Lift+Cruise Control/BASELINE_L1/Baseline/Scheduled Parameters/Smart_Interpolation ==
  data: u input; u_out output
function u_out = fcn(u)

% This function is used to limit interpolation for three portions of the
% flight envelope: 1) Below zero knots, 2) After the end of transition
% (90 kts) and before cruise (100 knots) and 3) above the last trim map
% point (130 knots)

ft2kts = 0.3048/1852.0*3600; % Conversion factor of ft/sec to knots (derived from setUnits values)
kts2ft = 1/ft2kts; % Conversion factor from knots to ft/sec
if u < 0* kts2ft; % SimIn.Control.trim.UH(1)
    u_out = 0*kts2ft; % SimIn.Control.trim.UH(1);
% elseif u>90*kts2ft && u<100*kts2ft
%     u_out = 100*kts2ft;
elseif u>130*kts2ft % SimIn.Control.trim.UH(end)
    u_out = 130*kts2ft; % SimIn.Control.trim.UH(end)
else
    u_out = u;
end

== matlab function GenCtrl/Lift+Cruise Control/BASELINE_L1/allocation/MATLAB Function ==
  data: u_lon input; u output; eng_max input; eng_min input; act_max input; act_min input
function u = Limited_Allocation(u_lon, eng_max, eng_min, act_max, act_min)
u = Limited_Long_Cont_Alloc_U(u_lon, eng_max, eng_min, act_max, act_min);

== matlab function GenCtrl/Lift+Cruise Control/BASELINE_L1/Baseline/Longitudinal Control/MATLAB Function ==
  data: Ap input; Ki output; Bp input; C input; q input; rdiag input; Kx output
function [Ki, Kx] = rslqr_tunning_lon(Ap, Bp, C, q, rdiag)
%#codegen
% lqr는 코드 생성 미지원 → 시뮬 전용 호출로 지정
coder.extrinsic('lqr');

% ===== 고정 차원 명시 =====
Nx  = int32(4);   % x=[u,w,q,th]
Ni  = int32(2);   % 적분기 상태
Nu  = int32(11);  % 제어입력 [T1..T9, delf, dele]

% ===== 입력 차원 검증(시뮬 동안 assert로 잡음) =====
assert(isequal(size(Ap), [double(Nx) double(Nx)]));
assert(isequal(size(Bp), [double(Nx) double(Nu)]));
assert(isequal(size(C ), [double(Ni) double(Nx)]));
assert(isvector(q)    && numel(q)    == double(Ni+Nx));   % Q 6
assert(isvector(rdiag)&& numel(rdiag)== double(Nu));      % R 11

% ===== Q,R 및 확장 상태공간 구성 =====
Q = diag(q(:));            % 6x6
R = diag(rdiag(:));        % 11x11
Dv = zeros(double(Ni), double(Nu), 'like', Ap);

At = [ zeros(double(Ni),double(Ni),'like',Ap)   C; 
       zeros(double(Nx),double(Ni),'like',Ap)   Ap ];

Bt = [ Dv; Bp ];

% ===== 출력/중간행렬 크기 미리 고정 =====
Ki = zeros(double(Nu), double(Ni), 'like', Ap);     % 11x2
Kx = zeros(double(Nu), double(Nx), 'like', Ap);     % 11x4
Kc = zeros(double(Nu), double(Ni+Nx), 'like', Ap);  % 11x6

% ===== lqr 호출(시뮬 전용) → 고정크기 행렬에 복사 =====
Ktmp = lqr(At, Bt, Q, R);      % extrinsic 호출: mxArray
Kc(:,:) = Ktmp;                % 크기 고정 행렬에 대입

% ===== 이 부분이 중요: 전체 행렬에서 블록 분할 =====
Ki(:,:) = Kc(:, 1:double(Ni));                      % 11x2
Kx(:,:) = Kc(:, double(Ni)+1 : double(Ni+Nx));      % 11x4
end
